simulink model "float_core_ref"  (R2025b)
settings: Solver=FixedStepAuto  StartTime=0.0  StopTime=10.0  FixedStep=0.05  RelTol=1e-3
settings Model: Creator=david  LastModifiedBy=david
settings OptimizationCC: DefaultParameterBehavior=Inlined  EnhancedBackFolding=on  PassReuseOutputArgsAs=Individual arguments  ZeroExternalMemoryAtStartup=off  ZeroInternalMemoryAtStartup=off  OptimizeBlockOrder=speed  DifferentSizesBufferReuse=on  OptimizationCustomize=off  EfficientTunableParamExpr=on
settings DebuggingCC: ParameterTunabilityLossMsg=error
settings SFSimCC: MATLABDynamicMemAlloc=off
settings RTWCC: SystemTargetFile=ert.tlc  TemplateMakefile=ert_default_tmf  Description=Embedded Coder
settings CodeAppCC: ForceParamTrailComments=on  IgnoreCustomStorageClasses=off  OperatorAnnotations=on  SimulinkDataObjDesc=on  SFDataObjDesc=on  InsertBlockDesc=on
settings ERTTargetCC: ERTCustomFileTemplate=example_file_process.tlc  TargetLangStandard=C99 (ISO)  GenerateSampleERTMain=on

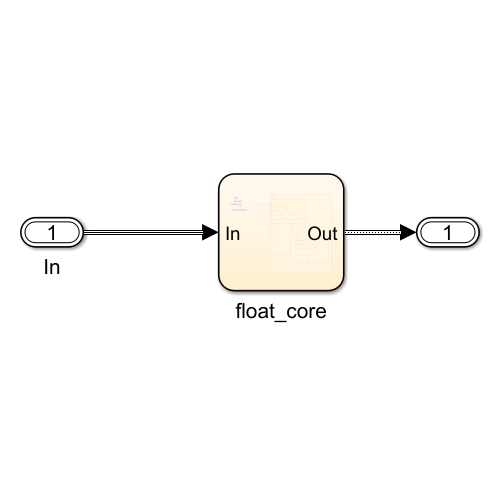
[thumbnail: Simulink's stored preview of the top-level diagram]
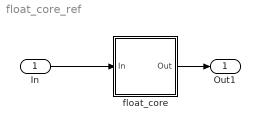
== system float_core_ref ==
  In : Inport  OutDataTypeStr=Bus: CoreInputsBus
  float_core : Stateflow chart  TreatAsAtomicUnit=on
  Out1 : Outport  OutDataTypeStr=Bus: CoreOutputsBus
  wires:
  In/1 -> float_core/1(In)
  float_core/1(Out) -> Out1/1

== stateflow chart float_core_ref/float_core ==
  state RUN
    state INIT
      during:
      reset_outputs();
      Out.led=int32(1);
    state HOMING
      during:
      reset_outputs();
      Out.led=int32(6);
      Out.motor_enable=true;
      st_home_t = st_home_t + double(In.dt_s);
      if st_home_t > P.homing_timeout_s
      req_safe=true;
      home_after=false;
      Out.motor_mode=int32(3);
      Out.log_now=true;
      Out.log_kind=int32(8);
      end
      state H_APPROACH
        during:
        Out.motor_mode=int32(2);
        Out.motor_target=int32(-1);   % JOG verso il TOF
        if In.tof_valid
        if In.tof_mm < P.tof_homing_approach_mm, home_confirm=home_confirm+uint8(1);
        else, home_confirm=uint8(0); end
        end
      state H_BACKOFF
        during:
        Out.motor_mode=int32(1);
        Out.motor_target=int32(last_cmd_target);
      state H_RETRACT
        during:
        Out.motor_mode=int32(2); Out.motor_target=int32(1);    % JOG via dal TOF
        if In.tof_valid
        if In.tof_mm > P.tof_homing_threshold_mm, home_confirm=home_confirm+uint8(1);
        else, home_confirm=uint8(0); end
        end
      (default) -> H_APPROACH
      H_APPROACH -> H_RETRACT : [home_confirm >= P.tof_homing_confirm_samples]{home_confirm=uint8(0); Out.motor_mode=int32(3);}
      H_RETRACT -> H_BACKOFF : [home_confirm >= P.tof_homing_confirm_samples]
          | {home_confirm=uint8(0); last_cmd_target=double(In.motor_pos)+double(P.endstop_margin_steps);
          | Out.motor_mode=int32(3);}
    state MISSION
      state M_PRE_DESCEND
        during:
        reset_outputs();
        Out.mission_active=true;
        Out.phase=int32(1);
        Out.led=int32(7);
        Out.log_now=true;
        Out.log_kind=int32(1);   % DEPLOY
      state M_DESCEND
        entry:  pid_phase_enter(true);
        during:
        reset_outputs();
        Out.mission_active=true;
        Out.phase=int32(2);
        phase_r = pid_phase(double(P.descent_target_m), double(P.hold_time_s), ...
        double(P.descent_timeout_s), true);
      state M_ASCEND
        entry:
        pid_phase_enter(false);
        during:
        reset_outputs();
        Out.mission_active=true;
        Out.phase=int32(3);
        phase_r = pid_phase(double(P.ascent_target_bottom_m), double(P.hold_time_s), double(P.ascent_timeout_s), true);
      state M_REST
        entry:
        pid_phase_enter(false);
        during:
        reset_outputs();
        Out.mission_active=true;
        Out.phase=int32(4);
        phase_r = pid_phase(double(P.rest_target_bottom_m), double(P.hold_time_s), ...
        double(P.rest_window_s), false);
      (default) -> M_PRE_DESCEND
      M_PRE_DESCEND -> M_DESCEND : [after(1,tick)]
      M_DESCEND -> M_ASCEND : [phase_r~=0]
      M_ASCEND -> M_DESCEND [order 1] : [phase_r~=0 && (st_completed+1) < P.profile_count]
          | { st_completed = st_completed + uint8(1); }
      M_ASCEND -> M_REST [order 2] : [phase_r~=0]
          | { st_completed = st_completed + uint8(1); }
    state IDLE
      entry:  req_safe=false;
      during:
      reset_outputs();
      if In.has_stored_data,
      Out.led=int32(3);
      else, Out.led=int32(2);
      end
      st_phase_t = st_phase_t + double(In.dt_s);
      if st_phase_t >= 0.5
      st_phase_t = 0;
      if In.has_stored_data, Out.ack_event=int32(5);
      else, Out.ack_event=int32(4); end
      end
    (default) -> INIT
    INIT -> HOMING : { st_home_t=0; home_confirm=uint8(0); }
    H_BACKOFF -> IDLE : [~In.motor_busy]{Out.motor_zero_here=true; Out.log_now=true; Out.log_kind=int32(8);}
    IDLE -> HOMING [order 2] : [In.event==2]
    IDLE -> MISSION [order 1] : [In.event==1]
    M_REST -> IDLE : [phase_r==2]
  state SAFE_STOP
    during:
    reset_outputs();
    Out.led=int32(4);
    Out.motor_mode=int32(3);
    Out.motor_enable=false;
  (default) -> RUN
  SAFE_STOP -> HOMING : [home_after || In.event==2]
      | { home_after=false;
      | st_home_t=0;
      | home_confirm=uint8(0); }
  RUN -> SAFE_STOP [order 1] : [In.event==3]
      | { Out.ack_event=int32(3);
      | Out.motor_mode=int32(3);
      | Out.led=int32(4);
      | Out.log_now=true;
      | Out.log_kind=int32(7);
      | home_after=false; }
  RUN -> SAFE_STOP [order 2] : [req_safe]
      | { req_safe=false; }
  data: u function_input; pos function_output; target function_input; u function_output; depth function_input; em function_output; with_kick function_input; target function_input; hold_s function_input; timeout_s function_input; exit_on_hold function_input; r function_output; Out output Bus: CoreOutputsBus; st_phase_t local double size=1 =0; st_home_t local double size=1 =0; home_after local boolean size=1 =false; In input Bus: CoreInputsBus; P parameter Bus: CoreConfigBus; req_safe local boolean size=1 =false; home_confirm local uint8 size=1 =0; st_completed local uint8 size=1 =0; last_cmd_target local double size=1 =0; st_stable_t local double size=1 =0; st_log_t local double size=1 =0; pid_integral local double size=1 =0; pid_dfilt local double size=1 =0; pid_last_depth local double size=1 =0; pid_has_last local boolean size=1 =false; at_ext_limit local boolean size=1 =false; tof_oor local uint8 size=1 =0; phase_r local double size=1 =0
  function reset_outputs:
    | function reset_outputs()
    |     % Default di ogni tick: chiamala per PRIMA in ogni entry: e during:.
    |     Out.motor_mode = int32(0);              % HOLD
    |     Out.motor_target = In.motor_pos;        % HOLD mantiene il target agganciato
    |     Out.motor_enable = false;
    |     Out.motor_zero_here = false;
    |     Out.led = int32(0);
    |     Out.phase = int32(0);
    |     Out.ack_event = int32(0);
    |     Out.log_now = false;
    |     Out.log_kind = int32(0);
    |     Out.mission_active = false;
    |     Out.completed_profiles = st_completed;
    | end
  function pos = u_to_pos(u):
    | function pos = u_to_pos(u)
    |     pos = int32(-round(u * double(P.usable_steps)));
    | end
  function pid_reset:
    | function pid_reset()
    |     pid_integral = 0; pid_dfilt = 0; pid_last_depth = 0; pid_has_last = false;
    | end
  function u = pid_compute(target, depth):
    | function u = pid_compute(target, depth)
    |     dt = double(In.dt_s);
    |     if dt <= 0 || dt > 1, dt = double(P.pid_period_s); end
    |     e = target - depth;
    |     P_ = double(P.kp) * e;
    |     if pid_has_last, dRaw = (depth - pid_last_depth)/dt; else, dRaw = 0; end
    |     pid_dfilt = double(P.alpha_d)*dRaw + (1-double(P.alpha_d))*pid_dfilt;
    |     D_ = -double(P.kd)*pid_dfilt;
    |     I_ = double(P.ki)*pid_integral;
    |     uRaw = double(P.u_neutral) + P_ + I_ + D_;
    |     u = min(1, max(0, uRaw));
    |     satHigh = uRaw > 1; satLow = uRaw < 0;
    |     if ~((satHigh && e > 0) || (satLow && e < 0))
    |         pid_integral = pid_integral + e*dt;
    |         pid_integral = min(double(P.integral_limit), max(-double(P.integral_limit), pid_integral));
    |     end
    |     pid_last_depth = depth; pid_has_last = true;
    | end
  function em = safety:
    | function em = safety()
    |     % Supervisore TOF (attivo solo in MISSION). Ritorna true su emergency.
    |     em = false;
    |     if ~In.tof_valid, return; end
    |     tooClose = In.tof_mm < P.tof_safe_min_mm;
    |     tooFar   = In.tof_mm > P.tof_safe_max_mm;
    |     if ~tooClose && ~tooFar, tof_oor = uint8(0); return; end
    |     tof_oor = tof_oor + uint8(1);
    |     if tof_oor < P.tof_safety_stop_samples, return; end
    |     tof_oor = uint8(0);
    |     if tooClose
    |         at_ext_limit = true; last_cmd_target = double(In.motor_pos);
    |         Out.motor_mode = int32(3); return;      % STOP pulito, inibisci estensione
    |     end
    |     req_safe = true; home_after = true;          % anomalia -> SAFE_STOP + auto-recovery
    |     Out.motor_mode = int32(3); Out.motor_enable = false;
    |     Out.led = int32(4); Out.log_now = true; Out.log_kind = int32(7);
    |     em = true;
    | end
  function pid_phase_enter(with_kick):
    | function pid_phase_enter(with_kick)
    |     pid_reset();
    |     phase_r = 0;                    % <-- AGGIUNGI: azzera l'esito fase all'ingresso
    |     st_phase_t = 0; st_stable_t = 0; st_log_t = 0;
    |     at_ext_limit = false; last_cmd_target = double(In.motor_pos);
    |     Out.led = int32(7); Out.motor_enable = true;
    |     if with_kick
    |         Out.motor_mode = int32(1);
    |         Out.motor_target = u_to_pos(double(P.descent_kick_u));
    |         last_cmd_target = double(Out.motor_target);
    |     end
    | end
  function r = pid_phase(target, hold_s, timeout_s, exit_on_hold):
    | function r = pid_phase(target, hold_s, timeout_s, exit_on_hold)
    |     r = 0;
    |     Out.led = int32(7); Out.motor_enable = true;
    |     if safety(), return; end                              % emergency: req_safe settato
    |     u = min(double(P.u_max), max(double(P.u_min), pid_compute(target, double(In.depth_m))));
    |     posTarget = double(u_to_pos(u));
    |     deadband  = double(P.min_retarget_frac) * double(P.usable_steps);
    |     retreating = posTarget > double(In.motor_pos);
    |     if (~at_ext_limit || retreating) && abs(posTarget - last_cmd_target) >= deadband
    |         Out.motor_mode = int32(1); Out.motor_target = int32(posTarget);
    |         last_cmd_target = posTarget; at_ext_limit = false;
    |     end
    |     if abs(double(In.depth_m) - target) < double(P.depth_tolerance_m)
    |         st_stable_t = st_stable_t + double(In.dt_s);
    |     else
    |         st_stable_t = 0;
    |     end
    |     st_log_t = st_log_t + double(In.dt_s);
    |     if st_log_t >= 1.0
    |         st_log_t = 0; Out.log_now = true; Out.log_kind = int32(2);  % PROFILE
    |     end
    |     st_phase_t = st_phase_t + double(In.dt_s);
    |     if exit_on_hold && st_stable_t >= hold_s, r = 1; return; end
    |     if st_phase_t >= timeout_s, r = 2; end
    | end
